simulink model "zad1"  (R2020b)
settings: Solver=FixedStepDiscrete  StartTime=0.0  StopTime=0.0  RelTol=1e-3
undefined symbols (not defined in the file): N3, N5, N7, P3, P5, P7
libraries: CPOiS_SourcesSinks x16, CPOiS_DataManipulation_DataTypeConversion x14, CPOiS_LinearTransforms x11, CPOiS_Filters x3, CPOiS_DataManipulation_IntroduceNoise x1, CPOiS_General x1
settings Model: Creator=jrybarz  LastModifiedBy=jrybarz

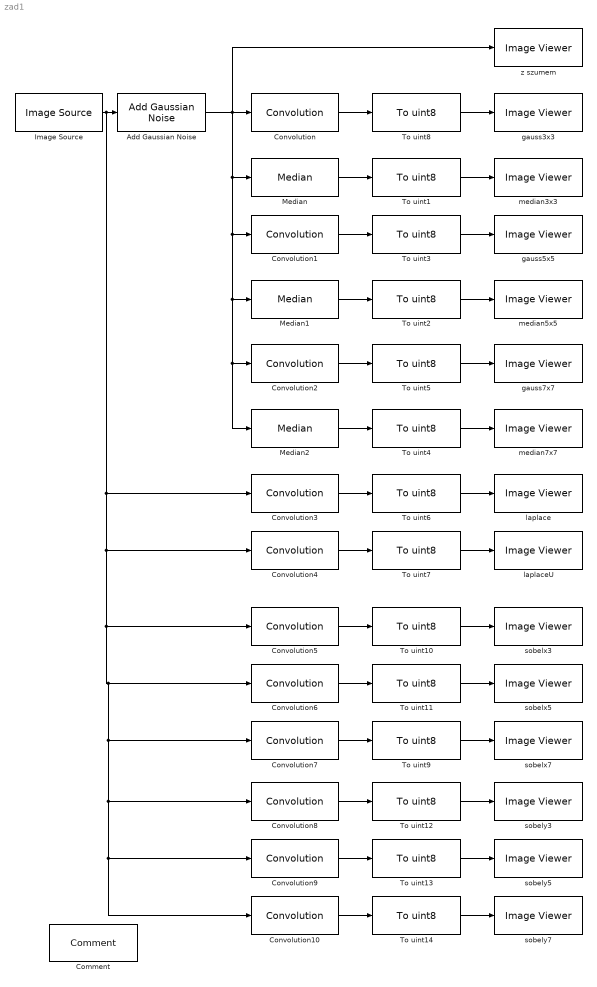
== system zad1 ==
  Add Gaussian Noise : CPOiS_DataManipulation_IntroduceNoise/Add Gaussian Noise  Mean=18.0  Variance=15.800
      settings: SourceProductName=CPOiS - Digital image and signal processing
  Comment : CPOiS_General/Comment
      settings: SourceProductName=CPOiS - Digital image and signal processing
  Convolution : CPOiS_LinearTransforms/Convolution  ConvolutionMatrix=[1,2,1;2,4,2;1,2,1]/16
      settings: SourceProductName=CPOiS - Digital image and signal processing
  Convolution1 : CPOiS_LinearTransforms/Convolution  ConvolutionMatrix=[1,4,6,4,1;4,16,24,16,4;6,24,36,24,6;4,16,24,16,4;1,4,6,4,1]/256
      settings: SourceProductName=CPOiS - Digital image and signal processing
  Convolution10 : CPOiS_LinearTransforms/Convolution  ConvolutionMatrix=P7*N7'
      settings: SourceProductName=CPOiS - Digital image and signal processing
  Convolution2 : CPOiS_LinearTransforms/Convolution  ConvolutionMatrix=(N7*N7')/4096
      settings: SourceProductName=CPOiS - Digital image and signal processing
  Convolution3 : CPOiS_LinearTransforms/Convolution  ConvolutionMatrix=[0,1,0;1,-4,1;0,1,0]
      settings: SourceProductName=CPOiS - Digital image and signal processing
  Convolution4 : CPOiS_LinearTransforms/Convolution  ConvolutionMatrix=[1,4,1;4,-20,4;1,4,1]/6
      settings: SourceProductName=CPOiS - Digital image and signal processing
  Convolution5 : CPOiS_LinearTransforms/Convolution  ConvolutionMatrix=N3*P3'
      settings: SourceProductName=CPOiS - Digital image and signal processing
  Convolution6 : CPOiS_LinearTransforms/Convolution  ConvolutionMatrix=N5*P5'
      settings: SourceProductName=CPOiS - Digital image and signal processing
  Convolution7 : CPOiS_LinearTransforms/Convolution  ConvolutionMatrix=N7*P7'
      settings: SourceProductName=CPOiS - Digital image and signal processing
  Convolution8 : CPOiS_LinearTransforms/Convolution  ConvolutionMatrix=P3*N3'
      settings: SourceProductName=CPOiS - Digital image and signal processing
  Convolution9 : CPOiS_LinearTransforms/Convolution  ConvolutionMatrix=P5*N5'
      settings: SourceProductName=CPOiS - Digital image and signal processing
  Image Source : CPOiS_SourcesSinks/Image Source  FileSelection=gull.png
      settings: SourceProductName=CPOiS - Digital image and signal processing
  Median : CPOiS_Filters/Median  MaskSize=3 x 3
      settings: SourceProductName=CPOiS - Digital image and signal processing
  Median1 : CPOiS_Filters/Median  MaskSize=5 x 5
      settings: SourceProductName=CPOiS - Digital image and signal processing
  Median2 : CPOiS_Filters/Median  MaskSize=7 x 7
      settings: SourceProductName=CPOiS - Digital image and signal processing
  To uint{1..14} (14 alike) : CPOiS_DataManipulation_DataTypeConversion/To uint8
      settings: SourceProductName=CPOiS - Digital image and signal processing
  gauss3x3 : CPOiS_SourcesSinks/Image Viewer
      settings: SourceProductName=CPOiS - Digital image and signal processing
  gauss5x5 : CPOiS_SourcesSinks/Image Viewer
      settings: SourceProductName=CPOiS - Digital image and signal processing
  gauss7x7 : CPOiS_SourcesSinks/Image Viewer
      settings: SourceProductName=CPOiS - Digital image and signal processing
  laplace : CPOiS_SourcesSinks/Image Viewer
      settings: SourceProductName=CPOiS - Digital image and signal processing
  laplaceU : CPOiS_SourcesSinks/Image Viewer
      settings: SourceProductName=CPOiS - Digital image and signal processing
  median3x3 : CPOiS_SourcesSinks/Image Viewer
      settings: SourceProductName=CPOiS - Digital image and signal processing
  median5x5 : CPOiS_SourcesSinks/Image Viewer
      settings: SourceProductName=CPOiS - Digital image and signal processing
  median7x7 : CPOiS_SourcesSinks/Image Viewer
      settings: SourceProductName=CPOiS - Digital image and signal processing
  sobelx3 : CPOiS_SourcesSinks/Image Viewer
      settings: SourceProductName=CPOiS - Digital image and signal processing
  sobelx5 : CPOiS_SourcesSinks/Image Viewer
      settings: SourceProductName=CPOiS - Digital image and signal processing
  sobelx7 : CPOiS_SourcesSinks/Image Viewer
      settings: SourceProductName=CPOiS - Digital image and signal processing
  sobely3 : CPOiS_SourcesSinks/Image Viewer
      settings: SourceProductName=CPOiS - Digital image and signal processing
  sobely5 : CPOiS_SourcesSinks/Image Viewer
      settings: SourceProductName=CPOiS - Digital image and signal processing
  sobely7 : CPOiS_SourcesSinks/Image Viewer
      settings: SourceProductName=CPOiS - Digital image and signal processing
  z szumem : CPOiS_SourcesSinks/Image Viewer
      settings: SourceProductName=CPOiS - Digital image and signal processing
  wires:
  Image Source/1 -> Convolution10/1, Convolution9/1, Convolution8/1, Convolution7/1, Convolution6/1, Convolution5/1, Convolution4/1, Convolution3/1, Add Gaussian Noise/1
  Median/1 -> To uint1/1
  To uint1/1 -> median3x3/1
  To uint8/1 -> gauss3x3/1
  Convolution/1 -> To uint8/1
  To uint3/1 -> gauss5x5/1
  Convolution1/1 -> To uint3/1
  Median1/1 -> To uint2/1
  To uint2/1 -> median5x5/1
  To uint4/1 -> median7x7/1
  To uint5/1 -> gauss7x7/1
  Add Gaussian Noise/1 -> z szumem/1, Median2/1, Convolution2/1, Median1/1, Convolution1/1, Median/1, Convolution/1
  Median2/1 -> To uint4/1
  Convolution2/1 -> To uint5/1
  To uint6/1 -> laplace/1
  Convolution3/1 -> To uint6/1
  Convolution4/1 -> To uint7/1
  To uint7/1 -> laplaceU/1
  To uint11/1 -> sobelx5/1
  Convolution6/1 -> To uint11/1
  Convolution5/1 -> To uint10/1
  To uint10/1 -> sobelx3/1
  To uint9/1 -> sobelx7/1
  Convolution7/1 -> To uint9/1
  To uint13/1 -> sobely5/1
  Convolution8/1 -> To uint12/1
  Convolution10/1 -> To uint14/1
  To uint12/1 -> sobely3/1
  To uint14/1 -> sobely7/1
  Convolution9/1 -> To uint13/1
